simulink library "BAT_cl"  (R2018b)
settings: Solver=VariableStepAuto  StartTime=0.0  StopTime=10.0  RelTol=1e-3
libraries: planarBAT_ul x1, planarTether_ul x1, simpleWinch_ul x1
settings Model: Creator=Ayaz  LastModifiedBy=Ayaz

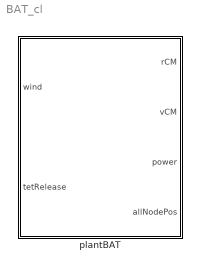
== system BAT_cl ==
  plantBAT : Subsystem  mask{rhoF=1, gravAcc=9.81, mT=1, BF=1.5, Sref=1, Cd=0.5, numNode=3, tetDia=0.001, tetDensity=1000, tetCD=0.5, tetYoungs=4e9, tetZeta=0.05, ini_rCM=[0;100], ini_vCM=[0;0], gndNodePos=[0;0], iniLength=0, maxRelease=0, maxTug=0}
      mask prompts: rhoF "Fluid density"; gravAcc "Gravitational acceleration"; mT "Mass"; BF "Buoyancy factor"; Sref "Reference area"; Cd "Drag coefficient"; numNode "Number of nodes"; tetDia "Tether diameter"; tetDensity "Tether density"; tetCD "Tether CD"; tetYoungs "Tether Young's modulus"; tetZeta "Tether damping ratio"; ini_rCM "Initial position"; ini_vCM "Initial velocity"; gndNodePos "Ground node position vector"; iniLength "Tether initial length"; maxRelease "Winch max release speed"; maxTug "Winch max tug speed"
      mask TypeOptions rhoF: planarBAT/rhoF | planarTether/rhoF
      mask TypeOptions gravAcc: planarBAT/gravAcc | planarTether/gravAcc
      mask TypeOptions mT: planarBAT/mT | planarTether/mT
      mask TypeOptions BF: planarBAT/BF
      mask TypeOptions Sref: planarBAT/Sref
      mask TypeOptions Cd: planarBAT/Cd
      mask TypeOptions numNode: planarTether/numNode
      mask TypeOptions tetDia: planarTether/tetDia
      mask TypeOptions tetDensity: planarTether/tetDensity
      mask TypeOptions tetCD: planarTether/tetCD
      mask TypeOptions tetYoungs: planarTether/tetYoungs
      mask TypeOptions tetZeta: planarTether/tetZeta
      mask TypeOptions maxRelease: simpleWinch/maxRelease
      mask TypeOptions maxTug: simpleWinch/maxTug
      mask DialogControl ParameterGroupVar Prompt: Environment
      mask DialogControl Container3 Prompt: Body
      mask DialogControl Container4 Prompt: Tether
      mask DialogControl Container5 Prompt: Initial conditions
      mask DialogControl Container6 Prompt: Winch

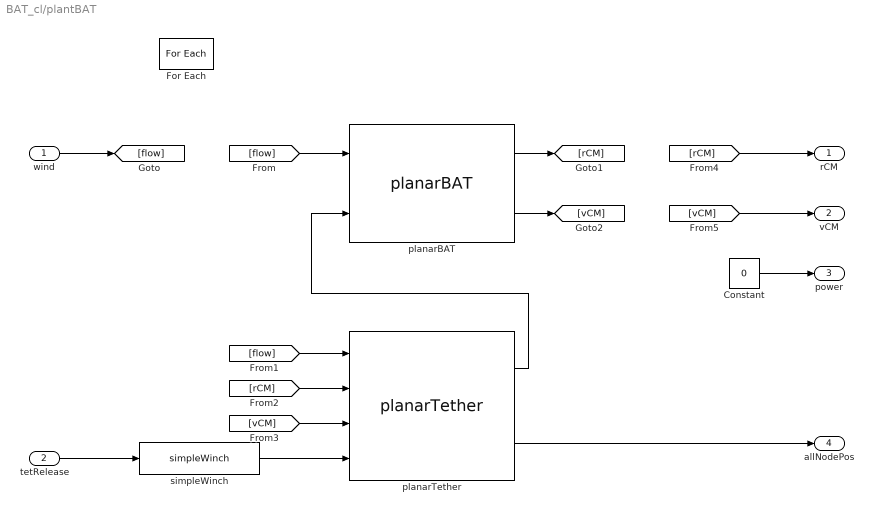
== system BAT_cl/plantBAT ==
  wind : Inport  Partition=on  PartitionDimension=2  PartitionWidth=1  PartitionOffset=0
  tetRelease : Inport  Port=2  Partition=on  PartitionDimension=2  PartitionWidth=1  PartitionOffset=0
  Constant : Constant  Value=0
  For Each : ForEach  DisableCoverage=on  IterateSubsysMaskParameter=off,off,off,off,off,off,off,off,off,off,off,off,on,on,on,on,off,off  SubsysMaskParameterIterationDimension=1,1,1,1,1,1,1,1,1,1,1,1,2,2,2,2,1,1  IndexMode=One-based
  planarBAT : planarBAT_ul/planarBAT  rhoF=rhoF  gravAcc=gravAcc  mT=mT  BF=BF  Sref=Sref  Cd=Cd  ini_rCM=ini_rCM  ini_vCM=ini_vCM
  planarTether : planarTether_ul/planarTether  rhoF=rhoF  gravAcc=gravAcc  numNode=numNode  tetDia=tetDia  tetDensity=tetDensity  tetCD=tetCD  tetYoungs=tetYoungs  tetZeta=tetZeta  mT=mT  gndNodePos=gndNodePos
  simpleWinch : simpleWinch_ul/simpleWinch  maxRelease=maxRelease  maxTug=maxTug  iniLength=iniLength
  rCM : Outport  ConcatenationDimension=2
  vCM : Outport  Port=2  ConcatenationDimension=2
  power : Outport  Port=3  ConcatenationDimension=2
  allNodePos : Outport  Port=4  ConcatenationDimension=3
  wires:
  wind/1 -> [flow]
  Constant/1 -> power/1
  [flow] -> planarBAT/1
  [flow] -> planarTether/1
  planarBAT/1 -> [rCM]
  planarBAT/2 -> [vCM]
  [rCM] -> planarTether/2
  [vCM] -> planarTether/3
  tetRelease/1 -> simpleWinch/1
  simpleWinch/1 -> planarTether/4
  planarTether/1 -> planarBAT/2
  planarTether/2 -> allNodePos/1
  [rCM] -> rCM/1
  [vCM] -> vCM/1
